simulink model "EventsOrder"  (Simulink 8.7)
settings: Solver=FixedStepDiscrete  StartTime=0.0  StopTime=51.0  RelTol=1e-3
settings Model: Creator=scaife  LastModifiedBy=bourbouh  ExtModeAutoUpdateStatusClock=off
settings DataIOCC: SignalLoggingSaveFormat=ModelDataLogs  SignalLoggingName=sigsOut
settings OptimizationCC: DefaultParameterBehavior=Inlined
settings DebuggingCC: AlgebraicLoopMsg=error  SaveWithParameterizedLinksMsg=none  SignalResolutionControl=TryResolveAllWithWarning  MultiTaskDSMMsg=warning  MultiTaskCondExecSysMsg=none
settings HardwareCC: ProdBitPerPointer=64  ProdLargestAtomicFloat=Float  ProdIntDivRoundTo=Zero  ProdEndianess=LittleEndian  ProdWordSize=64  ProdHWDeviceType=Intel->x86-64 (Windows64)  TargetBitPerLong=64  TargetBitPerPointer=64  TargetLongLongMode=on  TargetIntDivRoundTo=Zero  TargetEndianess=LittleEndian  TargetWordSize=64  TargetHWDeviceType=MATLAB Host  ProdEqTarget=off
settings SFSimCC: SimParseCustomCode=off
settings RTWCC: SystemTargetFile=rsim.tlc  TemplateMakefile=rsim_default_tmf  Description=Rapid Simulation Target  GenerateReport=on  LaunchReport=on  RTWCompilerOptimization=on
settings CodeAppCC: ForceParamTrailComments=on  OperatorAnnotations=on  MATLABSourceComments=on
settings RSimTargetCC: ERTMultiwordTypeDef=System defined  ERTMultiwordLength=256  GeneratePreprocessorConditionals=Use local settings

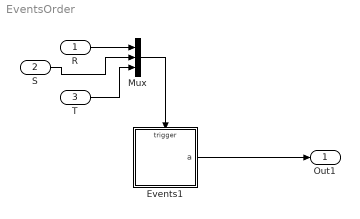
== system EventsOrder ==
  R : Inport
  S : Inport  Port=2
  T : Inport  Port=3
  Events1 : Stateflow chart  TreatAsAtomicUnit=on  RTWFileName=EventsOrder_code
      settings: RTWFileNameOpts=User specified
  Mux : Mux  Inputs=3
  Out1 : Outport
  wires:
  Events1/1(a) -> Out1/1
  Mux/1 -> Events1/Trigger
  R/1 -> Mux/1
  T/1 -> Mux/3
  S/1 -> Mux/2

== stateflow chart Events1 ==
  state A [parallel]
    settings: executionOrder=1
    state A2
      state A2a/
        en:a=a+3
      state A2b/
        en:a=a+4
      (default) -> A2a
      A2a -> A2b : S
      A2b -> A2a : R
    state A1
      state A1a/
        en:a=a+1
      state A1b/
        en:a=a+2
      (default) -> A1a
      A1a -> A1b : S
      A1b -> A1a : R
    (default) -> A1
    A1 -> A2 : T
    A2 -> A1 : T
  data: a output int32
  events: R input EITHER_EDGE_EVENT; S input EITHER_EDGE_EVENT; T input EITHER_EDGE_EVENT
